simulink model "expr1_1"  (R2021b)
settings: Solver=VariableStepAuto  StartTime=0.0  StopTime=50.0  RelTol=1e-3
settings Model: Creator=86137  LastModifiedBy=86137

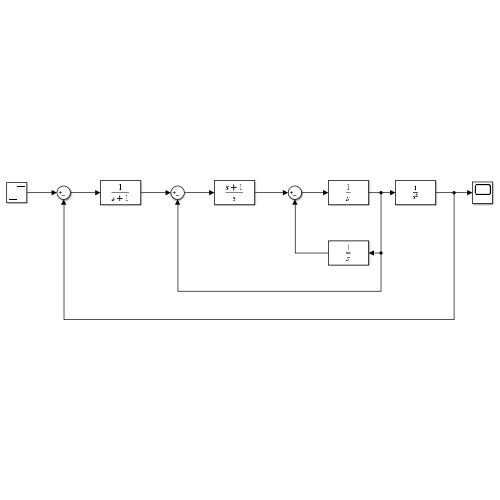
[thumbnail: Simulink's stored preview of the top-level diagram]
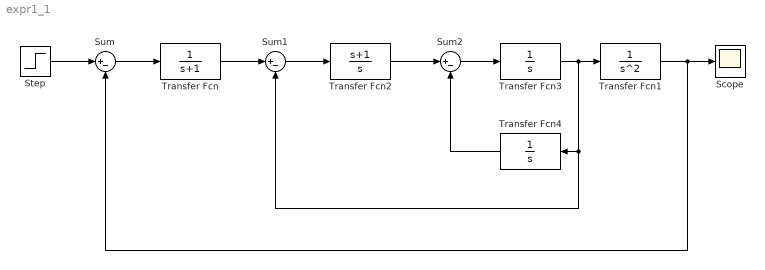
== system expr1_1 ==
  Scope : Scope
  Step : Step  SampleTime=0
  Sum : Sum  Inputs=|+-
  Sum1 : Sum  Inputs=|+-
  Sum2 : Sum  Inputs=|+-
  Transfer Fcn : TransferFcn  Denominator=[1 1]
  Transfer Fcn1 : TransferFcn  Denominator=[1 0 0]
  Transfer Fcn2 : TransferFcn  Numerator=[1 1]  Denominator=[1 0]
  Transfer Fcn3 : TransferFcn  Denominator=[1 0]
  Transfer Fcn4 : TransferFcn  Denominator=[1 0]
  wires:
  Sum/1 -> Transfer Fcn/1
  Transfer Fcn/1 -> Sum1/1
  Step/1 -> Sum/1
  Transfer Fcn1/1 -> Sum/2, Scope/1
  Sum1/1 -> Transfer Fcn2/1
  Transfer Fcn2/1 -> Sum2/1
  Sum2/1 -> Transfer Fcn3/1
  Transfer Fcn3/1 -> Transfer Fcn4/1, Sum1/2, Transfer Fcn1/1
  Transfer Fcn4/1 -> Sum2/2
